simulink model "Worked_Example_4_3"  (R2024b)
settings: Solver=VariableStepAuto  StartTime=0.0  StopTime=30  RelTol=1e-3
settings Model: Creator=GH-X-ST  LastModifiedBy=GH-X-ST

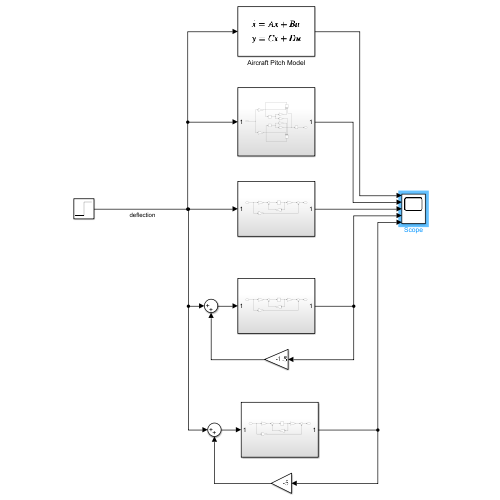
[thumbnail: Simulink's stored preview of the top-level diagram]
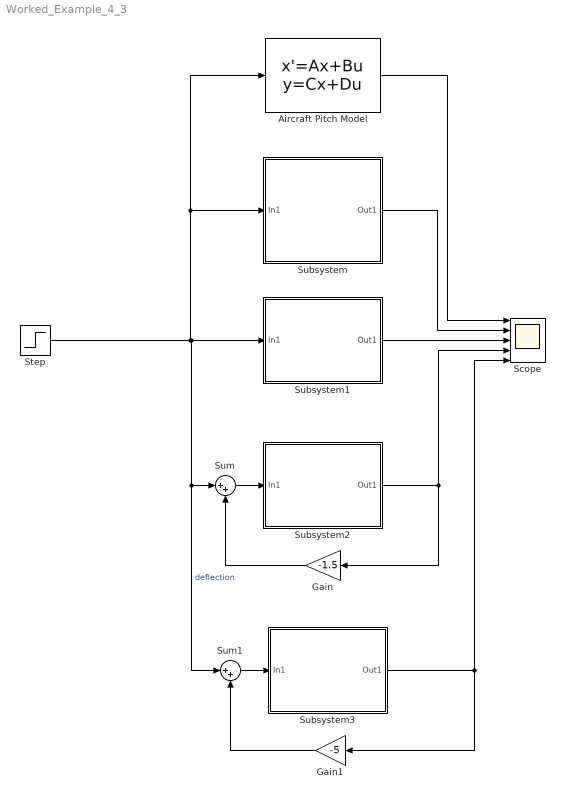
== system Worked_Example_4_3 ==
  Aircraft Pitch Model : StateSpace  A=[-0.3,57,0;-0.01,-0.5,0;0,57,0]  B=[0.232;0.0203;0]  C=[0,0,1]  D=[0]  InitialCondition=0  ContinuousStateAttributes='Aircraft_Pitch_Model'
  Gain : Gain  Gain=-1.5
  Gain1 : Gain  Gain=-5
  Scope : Scope  NumInputPorts=5
  Step : Step  SampleTime=0
  Subsystem : Subsystem
  Subsystem1 : Subsystem
  Subsystem2 : Subsystem
  Subsystem3 : Subsystem
  Sum : Sum  Inputs=|++
  Sum1 : Sum  Inputs=|++
  wires:
  Step/1 -> Subsystem1/1(In1), Sum1/1, Sum/1, Aircraft Pitch Model/1, Subsystem/1(In1)  "deflection"
  Aircraft Pitch Model/1 -> Scope/1
  Subsystem/1(Out1) -> Scope/2
  Subsystem2/1(Out1) -> Scope/4, Gain/1
  Subsystem1/1(Out1) -> Scope/3
  Gain/1 -> Sum/2
  Sum/1 -> Subsystem2/1(In1)
  Sum1/1 -> Subsystem3/1(In1)
  Subsystem3/1(Out1) -> Scope/5, Gain1/1
  Gain1/1 -> Sum1/2

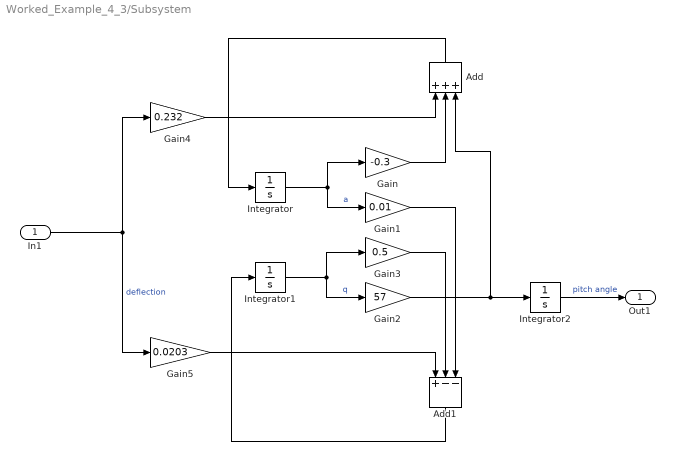
== system Worked_Example_4_3/Subsystem ==
  In1 : Inport
  Add : Sum  Inputs=+++
  Add1 : Sum  Inputs=+--
  Gain : Gain  Gain=-0.3
  Gain1 : Gain  Gain=0.01
  Gain2 : Gain  Gain=57
  Gain3 : Gain  Gain=0.5
  Gain4 : Gain  Gain=0.232
  Gain5 : Gain  Gain=0.0203
  Integrator : Integrator
  Integrator1 : Integrator
  Integrator2 : Integrator
  Out1 : Outport
  wires:
  Add1/1 -> Integrator1/1
  Gain5/1 -> Add1/1
  Add/1 -> Integrator/1
  Gain2/1 -> Integrator2/1, Add/3
  Integrator1/1 -> Gain3/1, Gain2/1  "q"
  Gain4/1 -> Add/1
  Gain/1 -> Add/2
  Gain1/1 -> Add1/3
  In1/1 -> Gain4/1, Gain5/1  "deflection"
  Integrator2/1 -> Out1/1  "pitch angle"
  Integrator/1 -> Gain/1, Gain1/1  "a"
  Gain3/1 -> Add1/2

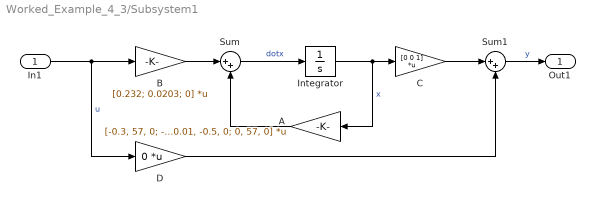
== system Worked_Example_4_3/Subsystem1 ==
  In1 : Inport
  A : Gain  Gain=[-0.3, 57, 0; -0.01, -0.5, 0; 0, 57, 0]  Multiplication=Matrix(K*u)
  B : Gain  Gain=[0.232; 0.0203; 0]  Multiplication=Matrix(K*u)
  C : Gain  Gain=[0 0 1]  Multiplication=Matrix(K*u)
  D : Gain  Gain=0  Multiplication=Matrix(K*u)
  Integrator : Integrator
  Sum : Sum  Inputs=|++
  Sum1 : Sum  Inputs=|++
  Out1 : Outport
  wires:
  In1/1 -> D/1, B/1  "u"
  Integrator/1 -> A/1, C/1  "x"
  A/1 -> Sum/2
  B/1 -> Sum/1
  Sum/1 -> Integrator/1  "dotx"
  C/1 -> Sum1/1
  D/1 -> Sum1/2
  Sum1/1 -> Out1/1  "y"

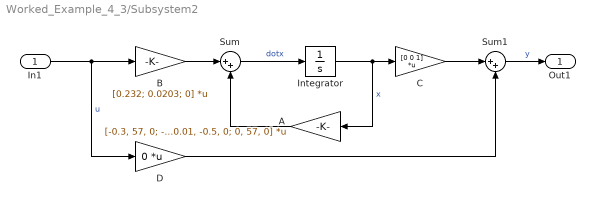
== system Worked_Example_4_3/Subsystem2 ==
  In1 : Inport
  A : Gain  Gain=[-0.3, 57, 0; -0.01, -0.5, 0; 0, 57, 0]  Multiplication=Matrix(K*u)
  B : Gain  Gain=[0.232; 0.0203; 0]  Multiplication=Matrix(K*u)
  C : Gain  Gain=[0 0 1]  Multiplication=Matrix(K*u)
  D : Gain  Gain=0  Multiplication=Matrix(K*u)
  Integrator : Integrator
  Sum : Sum  Inputs=|++
  Sum1 : Sum  Inputs=|++
  Out1 : Outport
  wires:
  In1/1 -> D/1, B/1  "u"
  Integrator/1 -> A/1, C/1  "x"
  A/1 -> Sum/2
  B/1 -> Sum/1
  Sum/1 -> Integrator/1  "dotx"
  C/1 -> Sum1/1
  D/1 -> Sum1/2
  Sum1/1 -> Out1/1  "y"

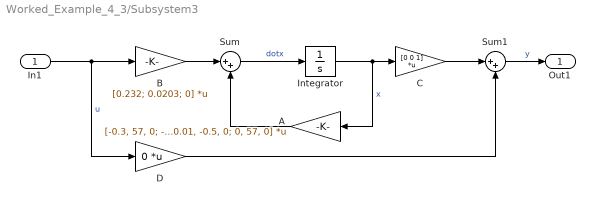
== system Worked_Example_4_3/Subsystem3 ==
  In1 : Inport
  A : Gain  Gain=[-0.3, 57, 0; -0.01, -0.5, 0; 0, 57, 0]  Multiplication=Matrix(K*u)
  B : Gain  Gain=[0.232; 0.0203; 0]  Multiplication=Matrix(K*u)
  C : Gain  Gain=[0 0 1]  Multiplication=Matrix(K*u)
  D : Gain  Gain=0  Multiplication=Matrix(K*u)
  Integrator : Integrator
  Sum : Sum  Inputs=|++
  Sum1 : Sum  Inputs=|++
  Out1 : Outport
  wires:
  In1/1 -> D/1, B/1  "u"
  Integrator/1 -> A/1, C/1  "x"
  A/1 -> Sum/2
  B/1 -> Sum/1
  Sum/1 -> Integrator/1  "dotx"
  C/1 -> Sum1/1
  D/1 -> Sum1/2
  Sum1/1 -> Out1/1  "y"
